simulink model "x35BusNetworkElectricityTransmissionModel"  (R2023b)
settings: Solver=VariableStepAuto  StartTime=0.0  StopTime=0.8  RelTol=1e-3
model workspace (MAT data in the model file):
  Compensation_Ki = 30
  Compensation_Kp = 3
  DC_Ki = 400
  DC_Kp = 8
  F = 0.01
  Flux_min = 0.5
  Grid_Freq_PWM = 2700
  Grid_Ireg_Ki = 5
  Grid_Ireg_Kp = 0.83
  Grid_Ireg_lim = 1.1
  Grid_Modindex_Upper = 1.1
  Grid_conv_Imax = 0.8
  H = 0.685
  Idref_max = 0.9
  Iqref_Tc = 0.3
  Ki_Var = 0.05
  Ki_Vreg = 20
  Ksh = 1.1
  L_pu = 0.3
  Llr = 0.16
  Lls = 0.18
  Lm = 2.9
  Nb_wt = 6
  P_mech = 1080000
  Pitch_Ki = 0
  Pitch_Kp = 150
  Pitch_Max = 27
  Pitch_Tc = 0.01
  Pitch_rate = 10
  Q_Filt = 50
  R_pu = 0.003
  Rotor_Freq_PWM = 1620
  Rotor_Ireg_Ki = 8
  Rotor_Ireg_Kp = 0.6
  Rotor_Ireg_lim = 0.1
  Rotor_Modindex_Upper = 2
  Rr = 0.016
  Rs = 0.023
  T_set = 0.0001
  Tp = 5e-05
  Ts = 5e-06
  Var_C_Filt = 720000
  Var_reg_max = 1.1
  Var_reg_min = 0.9
  WT_Coeff = [0.645 116 0.4 5 21 0.00912 0.08 0.035]
  WT_H = 4.32
  WT_IGBTRon = 5.931
  WT_Param = [91.204 10143]
  Wind_Freq_Filt = 10000
  Wind_Freq_nom = 60
  Wind_P_nom = 1200000
  Wind_Rotor_V_nom = 1950
  Wind_V_nom = 500
  Zeta_Filt = 0.707106781187
  init = [-0.2 0 0 0 0 0 0 0]
  p = 3
  torque0 = 0.83
  v_Ki = 0.1
  v_Kp = 3.6
  v_Max = 1.2
  v_Min = 0.7
  v_T = 5
  vreg_max = 1
  wind_VDC_nom = 1150
  wt0 = 1.2
undefined symbols (not defined in the file): D1, D11, Delta, DiscIntNeverNeededParam, Ion, Lithium, P, Q
libraries: powerlib_extras x144, spsSeriesRLCBranchLib x67, spsLoadFlowBusLib x43, spsThreePhaseTransformerTwoWindingsLib x32, spsThreePhaseSeriesRLCLoadLib x31, spsThreePhaseVIMeasurementLib x26, simulink_extras x26, spsDistributedParametersLineLib x22, spsGenericPowerSystemStabilizerLib x20, spsSynchronousMachinepuStandardLib x10, spsExcitationSystemLib x10, spsHydraulicTurbineandGovernorLib x10
(part 9 of 16)

== system x35BusNetworkElectricityTransmissionModel/ 41.4 MW Wind Generation/41.4 MW Wind Farm/Control System/Control System 4 ==
  Vabc : Inport
  Stator_Iabc : Inport  Port=2
  Grid_Iabc : Inport  Port=3
  Rotor_Iabc : Inport  Port=4
  Vdc_V : Inport  Port=5
  Qref1 : Inport  Port=6
  angle_rotor_rad : Inport  Port=7
  wr : Inport  Port=8
  Bus Creator : BusCreator  Inputs=P,Q
  Constant : Constant  Value=0
  Grid-side Control System : Subsystem
  "Measurement and abc-to-dq transformation " : Subsystem
  PWM Generator (2-Level) : spsPWMGenerator2LevelLib/PWM Generator (2-Level)  ModulatorType=Three-phase bridge (6 pulses)  ModulatorMode=Unsynchronized  Fc=Grid_Freq_PWM  Pc=90  nF=27  MinMax="[ -1  1 ]"  SamplingTechnique=Natural  ModulatingSignals=off  m=0.8  Freq=60  Phase=0  Ts=Ts  ShowCarrierOutport=off
  PWM Generator (2-Level)1 : spsPWMGenerator2LevelLib/PWM Generator (2-Level)  ModulatorType=Three-phase bridge (6 pulses)  ModulatorMode=Unsynchronized  Fc=Rotor_Freq_PWM  Pc=90  nF=27  MinMax="[ -1  1 ]"  SamplingTechnique=Natural  ModulatingSignals=off  m=0.8  Freq=60  Phase=0  Ts=Ts  ShowCarrierOutport=off
  Rotor-side Control System : Subsystem
  Speed & Pitch Control System : Subsystem
  Unit Delay{,2..5} (5 alike) : UnitDelay  SampleTime=Ts  HasFrameUpgradeWarning=on
  Grid_conv_pulses : Outport
  Rotor_conv_pulses : Outport  Port=2
  Pitch : Outport  Port=3
  PQ : Outport  Port=4
  wires:
  [Meas_P] -> Speed & Pitch Control System/2(Meas_P)
  "Measurement and abc-to-dq transformation "/1(Stator_Vdq) -> [Stator_Vdq]
  [Meas_Q] -> Unit Delay4/1
  Unit Delay4/1 -> Bus Creator/2  "Q"
  "Measurement and abc-to-dq transformation "/2(Stator_Idq) -> [Stator_Idq]
  "Measurement and abc-to-dq transformation "/9(w) -> [w]
  Grid_Iabc/1 -> "Measurement and abc-to-dq transformation "/3(Grid_Iabc)
  Grid-side Control System/1(Grid_conv_V) -> Unit Delay/1
  Unit Delay5/1 -> PWM Generator (2-Level)1/1
  Unit Delay2/1 -> Pitch/1
  Unit Delay/1 -> PWM Generator (2-Level)/1
  "Measurement and abc-to-dq transformation "/3(Grid_conv_Idq) -> [Grid_Idq]
  Rotor-side Control System/1(Uctrl_rotor_conv) -> Unit Delay5/1
  "Measurement and abc-to-dq transformation "/13(Delta_Rotor_Angle) -> [Delta_rotor_angle]
  PWM Generator (2-Level)/1 -> Grid_conv_pulses/1
  Vabc/1 -> "Measurement and abc-to-dq transformation "/1(Vabc)
  PWM Generator (2-Level)1/1 -> Rotor_conv_pulses/1
  "Measurement and abc-to-dq transformation "/4(Rotor_Idq) -> [Rotor_Idq]
  "Measurement and abc-to-dq transformation "/5(Vdc_meas_V) -> [Meas_VDC]
  angle_rotor_rad/1 -> "Measurement and abc-to-dq transformation "/7(angle_rotor_rad)
  wr/1 -> "Measurement and abc-to-dq transformation "/8(wr)
  "Measurement and abc-to-dq transformation "/7(Meas_Q) -> [Meas_Q]
  Speed & Pitch Control System/2(Pitch (deg)) -> Unit Delay2/1
  Stator_Iabc/1 -> "Measurement and abc-to-dq transformation "/2(Stator_Iabc)
  Speed & Pitch Control System/1(Tem_cmd) -> [Tem_cmd]
  Rotor_Iabc/1 -> "Measurement and abc-to-dq transformation "/4(Rotor_Iabc)
  Vdc_V/1 -> "Measurement and abc-to-dq transformation "/5(Vdc_V)
  Qref1/1 -> "Measurement and abc-to-dq transformation "/6(Qref)
  [wr] -> Speed & Pitch Control System/1(wr1)
  [Meas_P] -> Unit Delay3/1
  Unit Delay3/1 -> Bus Creator/1  "P"
  "Measurement and abc-to-dq transformation "/11("Qref ") -> [Q_ref]
  "Measurement and abc-to-dq transformation "/6(Meas_P) -> [Meas_P]
  "Measurement and abc-to-dq transformation "/12(Theta_PLL) -> [PLL_theta]
  Bus Creator/1 -> PQ/1
  "Measurement and abc-to-dq transformation "/8(Meas_V) -> [Meas_V]
  "Measurement and abc-to-dq transformation "/10("wr ") -> [wr]
  [Stator_Vdq] -> Grid-side Control System/1(Stator_Vdq)
  Constant/1 -> Grid-side Control System/2(Iq_ref)
  [Meas_VDC] -> Grid-side Control System/3(Vdc)
  [Grid_Idq] -> Grid-side Control System/4(Grid_conv_Idq)
  [PLL_theta] -> Grid-side Control System/5(Theta_PLL)
  [w] -> Grid-side Control System/6(w)
  [Rotor_Idq] -> Rotor-side Control System/1(Rotor_Idq)
  [wr] -> Rotor-side Control System/2(wr)
  [Meas_VDC] -> Rotor-side Control System/3(Vdc)
  [Delta_rotor_angle] -> Rotor-side Control System/4(Angle)
  [Q_ref] -> Rotor-side Control System/5(Qref)
  [Meas_Q] -> Rotor-side Control System/6(Meas_Q)
  [Meas_V] -> Rotor-side Control System/7(Meas_V)
  [Stator_Vdq] -> Rotor-side Control System/8(Stator_Vdq)
  [w] -> Rotor-side Control System/9(w)
  [Stator_Idq] -> Rotor-side Control System/10(Stator_Idq)
  [Tem_cmd] -> Rotor-side Control System/11(Tem_cmd)

== system x35BusNetworkElectricityTransmissionModel/400 kV Solar Farm/DC//DC Boost Converter/MPPT/MPPT  ==
  note: This model uses incremental conductance method to get maximum power point
      |
      | when dP/dV=0  where P= V*I
      | -> d(V*I)/dV = I + V*dI/dV = 0
      | -> dI/dV = -I/V
      |
      | The integrator functions to reduce/minimize errors (dI/dV + I/V)
      | Output = duty cycle changes
  PV_Current : Inport
  PV_Voltage : Inport  Port=2
  Switch port : Inport  Port=3
  Constant2 : Constant  Value=0
  Constant3 : Constant  Value=0
  Dead Zone : DeadZone  LowerValue=-0.05  UpperValue=0.05
  Discrete-Time Integrator : DiscreteIntegrator  SampleTime=T_set  LimitOutput=on  UpperSaturationLimit=1  LowerSaturationLimit=-1  ICPrevOutput=DiscIntNeverNeededParam  ICPrevScaledInput=DiscIntNeverNeededParam
  Fourier : spsFourierLib/Fourier  Freq=1/(MPPT_time)  n=1  InInit=[0, 0]  Ts=T_set
  Fourier1 : spsFourierLib/Fourier  Freq=1/(MPPT_time)  n=1  InInit=[0, 0]  Ts=T_set
  Gain : Gain  Gain=5
  Mean : spsMeanLib/Mean  Freq=1/(MPPT_time)  Vinit=0  Ts=T_set
  Mean1 : spsMeanLib/Mean  Freq=1/(MPPT_time)  Vinit=0  Ts=T_set
  Product : Product  Inputs=*/
  Product2 : Product
  Product3 : Product  Inputs=*/
  Saturation : Saturate  UpperLimit=inf  LowerLimit=eps  ZeroCross=off
  Saturation1 : Saturate  UpperLimit=inf  LowerLimit=eps  ZeroCross=off
  Sum : Sum  Inputs=+-
  Sum1 : Sum
  Switch : Switch  Threshold=0.5  SaturateOnIntegerOverflow=off  InputSameDT=off
  Switch1 : Switch  Threshold=0.5  SaturateOnIntegerOverflow=off  InputSameDT=off
  Trigonometric Function : Trigonometry  Operator=cos
  deg-to-rad conversion : Gain  Gain=pi/180
  delta D : Outport
  tag scope: Imean_PV1=global, Vmean_PV1=global
  wires:
  Mean1/1 -> [Vmean_PV1], Saturation1/1
  PV_Voltage/1 -> Mean1/1, Fourier1/1
  Sum/1 -> deg-to-rad conversion/1
  Product/1 -> Product2/1
  Product3/1 -> Sum1/2
  Saturation1/1 -> Product3/2
  Switch port/1 -> Switch/2, Switch1/2
  Mean/1 -> [Imean_PV1], Product3/1
  Dead Zone/1 -> Gain/1
  Fourier/2 -> Sum/1
  Fourier1/1 -> Saturation/1
  Sum1/1 -> Switch/1  "error"
  Constant2/1 -> Switch/3
  Trigonometric Function/1 -> Product2/2
  Gain/1 -> Discrete-Time Integrator/1
  Discrete-Time Integrator/1 -> Switch1/1
  Switch/1 -> Dead Zone/1
  Fourier1/2 -> Sum/2
  Constant3/1 -> Switch1/3
  deg-to-rad conversion/1 -> Trigonometric Function/1
  PV_Current/1 -> Mean/1, Fourier/1
  Product2/1 -> Sum1/1  "dI/dV (PV)"
  Saturation/1 -> Product/2
  Fourier/1 -> Product/1
  Switch1/1 -> delta D/1

== system x35BusNetworkElectricityTransmissionModel/400 kV Solar Farm/DC//DC Boost Converter1/MPPT/MPPT  ==
  note: This model uses incremental conductance method to get maximum power point
      |
      | when dP/dV=0  where P= V*I
      | -> d(V*I)/dV = I + V*dI/dV = 0
      | -> dI/dV = -I/V
      |
      | The integrator functions to reduce/minimize errors (dI/dV + I/V)
      | Output = duty cycle changes
  PV_Current : Inport
  PV_Voltage : Inport  Port=2
  Switch port : Inport  Port=3
  Constant2 : Constant  Value=0
  Constant3 : Constant  Value=0
  Dead Zone : DeadZone  LowerValue=-0.05  UpperValue=0.05
  Discrete-Time Integrator : DiscreteIntegrator  SampleTime=T_set  LimitOutput=on  UpperSaturationLimit=1  LowerSaturationLimit=-1  ICPrevOutput=DiscIntNeverNeededParam  ICPrevScaledInput=DiscIntNeverNeededParam
  Fourier : spsFourierLib/Fourier  Freq=1/(MPPT_time)  n=1  InInit=[0, 0]  Ts=T_set
  Fourier1 : spsFourierLib/Fourier  Freq=1/(MPPT_time)  n=1  InInit=[0, 0]  Ts=T_set
  Gain : Gain  Gain=5
  Mean : spsMeanLib/Mean  Freq=1/(MPPT_time)  Vinit=0  Ts=T_set
  Mean1 : spsMeanLib/Mean  Freq=1/(MPPT_time)  Vinit=0  Ts=T_set
  Product : Product  Inputs=*/
  Product2 : Product
  Product3 : Product  Inputs=*/
  Saturation : Saturate  UpperLimit=inf  LowerLimit=eps  ZeroCross=off
  Saturation1 : Saturate  UpperLimit=inf  LowerLimit=eps  ZeroCross=off
  Sum : Sum  Inputs=+-
  Sum1 : Sum
  Switch : Switch  Threshold=0.5  SaturateOnIntegerOverflow=off  InputSameDT=off
  Switch1 : Switch  Threshold=0.5  SaturateOnIntegerOverflow=off  InputSameDT=off
  Trigonometric Function : Trigonometry  Operator=cos
  deg-to-rad conversion : Gain  Gain=pi/180
  delta D : Outport
  tag scope: Imean_PV2=global, Vmean_PV2=global
  wires:
  Mean1/1 -> Saturation1/1
  PV_Voltage/1 -> Mean1/1, Fourier1/1
  Sum/1 -> deg-to-rad conversion/1
  Product/1 -> Product2/1
  Product3/1 -> Sum1/2
  Saturation1/1 -> [Vmean_PV2], Product3/2
  Switch port/1 -> Switch/2, Switch1/2
  Mean/1 -> [Imean_PV2], Product3/1
  Dead Zone/1 -> Gain/1
  Fourier/2 -> Sum/1
  Fourier1/1 -> Saturation/1
  Sum1/1 -> Switch/1  "error"
  Constant2/1 -> Switch/3
  Trigonometric Function/1 -> Product2/2
  Gain/1 -> Discrete-Time Integrator/1
  Discrete-Time Integrator/1 -> Switch1/1
  Switch/1 -> Dead Zone/1
  Fourier1/2 -> Sum/2
  Constant3/1 -> Switch1/3
  deg-to-rad conversion/1 -> Trigonometric Function/1
  PV_Current/1 -> Mean/1, Fourier/1
  Product2/1 -> Sum1/1  "dI/dV (PV)"
  Saturation/1 -> Product/2
  Fourier/1 -> Product/1
  Switch1/1 -> delta D/1

== system x35BusNetworkElectricityTransmissionModel/400 kV Solar Farm/DC//DC Boost Converter2/MPPT/MPPT  ==
  note: This model uses incremental conductance method to get maximum power point
      |
      | when dP/dV=0  where P= V*I
      | -> d(V*I)/dV = I + V*dI/dV = 0
      | -> dI/dV = -I/V
      |
      | The integrator functions to reduce/minimize errors (dI/dV + I/V)
      | Output = duty cycle changes
  PV_Current : Inport
  PV_Voltage : Inport  Port=2
  Switch port : Inport  Port=3
  Constant2 : Constant  Value=0
  Constant3 : Constant  Value=0
  Dead Zone : DeadZone  LowerValue=-0.05  UpperValue=0.05
  Discrete-Time Integrator : DiscreteIntegrator  SampleTime=T_set  LimitOutput=on  UpperSaturationLimit=1  LowerSaturationLimit=-1  ICPrevOutput=DiscIntNeverNeededParam  ICPrevScaledInput=DiscIntNeverNeededParam
  Display : Display
  Fourier : spsFourierLib/Fourier  Freq=1/(MPPT_time)  n=1  InInit=[0, 0]  Ts=T_set
  Fourier1 : spsFourierLib/Fourier  Freq=1/(MPPT_time)  n=1  InInit=[0, 0]  Ts=T_set
  Gain : Gain  Gain=5
  Mean : spsMeanLib/Mean  Freq=1/(MPPT_time)  Vinit=0  Ts=T_set
  Mean1 : spsMeanLib/Mean  Freq=1/(MPPT_time)  Vinit=0  Ts=T_set
  Product : Product  Inputs=*/
  Product2 : Product
  Product3 : Product  Inputs=*/
  Saturation : Saturate  UpperLimit=inf  LowerLimit=eps  ZeroCross=off
  Saturation1 : Saturate  UpperLimit=inf  LowerLimit=eps  ZeroCross=off
  Sum : Sum  Inputs=+-
  Sum1 : Sum
  Switch : Switch  Threshold=0.5  SaturateOnIntegerOverflow=off  InputSameDT=off
  Switch1 : Switch  Threshold=0.5  SaturateOnIntegerOverflow=off  InputSameDT=off
  Trigonometric Function : Trigonometry  Operator=cos
  deg-to-rad conversion : Gain  Gain=pi/180
  delta D : Outport
  tag scope: Imean_PV3=global, Vmean_PV3=global
  wires:
  Mean1/1 -> Saturation1/1
  PV_Voltage/1 -> Mean1/1, Fourier1/1
  Sum/1 -> deg-to-rad conversion/1
  Product/1 -> Product2/1
  Product3/1 -> Sum1/2
  Saturation1/1 -> [Vmean_PV3], Product3/2
  Switch port/1 -> Switch/2, Switch1/2
  Dead Zone/1 -> Gain/1
  Fourier/2 -> Sum/1
  Fourier1/1 -> Saturation/1
  Sum1/1 -> Switch/1  "error"
  Constant2/1 -> Switch/3
  Trigonometric Function/1 -> Product2/2
  Gain/1 -> Discrete-Time Integrator/1
  Discrete-Time Integrator/1 -> Switch1/1
  Switch/1 -> Dead Zone/1
  Fourier1/2 -> Sum/2
  Constant3/1 -> Switch1/3
  deg-to-rad conversion/1 -> Trigonometric Function/1
  PV_Current/1 -> Mean/1, Fourier/1
  Product2/1 -> Sum1/1  "dI/dV (PV)"
  Saturation/1 -> Product/2
  Fourier/1 -> Product/1
  Switch1/1 -> delta D/1
  Mean/1 -> Display/1, [Imean_PV3], Product3/1

== system x35BusNetworkElectricityTransmissionModel/400 kV Solar Farm/DC//DC Boost Converter3/MPPT/MPPT  ==
  note: This model uses incremental conductance method to get maximum power point
      |
      | when dP/dV=0  where P= V*I
      | -> d(V*I)/dV = I + V*dI/dV = 0
      | -> dI/dV = -I/V
      |
      | The integrator functions to reduce/minimize errors (dI/dV + I/V)
      | Output = duty cycle changes
  PV_Current : Inport
  PV_Voltage : Inport  Port=2
  Switch port : Inport  Port=3
  Constant2 : Constant  Value=0
  Constant3 : Constant  Value=0
  Dead Zone : DeadZone  LowerValue=-0.05  UpperValue=0.05
  Discrete-Time Integrator : DiscreteIntegrator  SampleTime=T_set  LimitOutput=on  UpperSaturationLimit=1  LowerSaturationLimit=-1  ICPrevOutput=DiscIntNeverNeededParam  ICPrevScaledInput=DiscIntNeverNeededParam
  Fourier : spsFourierLib/Fourier  Freq=1/(MPPT_time)  n=1  InInit=[0, 0]  Ts=T_set
  Fourier1 : spsFourierLib/Fourier  Freq=1/(MPPT_time)  n=1  InInit=[0, 0]  Ts=T_set
  Gain : Gain  Gain=5
  Mean : spsMeanLib/Mean  Freq=1/(MPPT_time)  Vinit=0  Ts=T_set
  Mean1 : spsMeanLib/Mean  Freq=1/(MPPT_time)  Vinit=0  Ts=T_set
  Product : Product  Inputs=*/
  Product2 : Product
  Product3 : Product  Inputs=*/
  Saturation : Saturate  UpperLimit=inf  LowerLimit=eps  ZeroCross=off
  Saturation1 : Saturate  UpperLimit=inf  LowerLimit=eps  ZeroCross=off
  Sum : Sum  Inputs=+-
  Sum1 : Sum
  Switch : Switch  Threshold=0.5  SaturateOnIntegerOverflow=off  InputSameDT=off
  Switch1 : Switch  Threshold=0.5  SaturateOnIntegerOverflow=off  InputSameDT=off
  Trigonometric Function : Trigonometry  Operator=cos
  deg-to-rad conversion : Gain  Gain=pi/180
  delta D : Outport
  tag scope: Imean_PV4=global, Vmean_PV4=global
  wires:
  Mean1/1 -> Saturation1/1
  PV_Voltage/1 -> Mean1/1, Fourier1/1
  Sum/1 -> deg-to-rad conversion/1
  Product/1 -> Product2/1
  Product3/1 -> Sum1/2
  Saturation1/1 -> [Vmean_PV4], Product3/2
  Switch port/1 -> Switch/2, Switch1/2
  Dead Zone/1 -> Gain/1
  Fourier/2 -> Sum/1
  Fourier1/1 -> Saturation/1
  Sum1/1 -> Switch/1  "error"
  Constant2/1 -> Switch/3
  Trigonometric Function/1 -> Product2/2
  Gain/1 -> Discrete-Time Integrator/1
  Discrete-Time Integrator/1 -> Switch1/1
  Switch/1 -> Dead Zone/1
  Fourier1/2 -> Sum/2
  Constant3/1 -> Switch1/3
  deg-to-rad conversion/1 -> Trigonometric Function/1
  PV_Current/1 -> Mean/1, Fourier/1
  Product2/1 -> Sum1/1  "dI/dV (PV)"
  Saturation/1 -> Product/2
  Fourier/1 -> Product/1
  Switch1/1 -> delta D/1
  Mean/1 -> [Imean_PV4], Product3/1

== system x35BusNetworkElectricityTransmissionModel/North Network/Regulators 7/Turbine and Excitation Regulators/Stabilitator ==
  Pm : Inport
  Pe : Inport  Port=2
  dw : Inport  Port=3
  Add1 : Sum  Inputs=+-
  Generic Power System Stabilizer : spsGenericPowerSystemStabilizerLib/Generic Power System Stabilizer  Tsensor=30e-3  K=20  Twashout=2  Tleadlag1=[50e-3 20e-3]  Tleadlag2=[3 5.4]  VSlimits=[-0.15 0.15]  Vinit=0  Plot_On=off  MagdB_On=on  FreqRange=logspace(-2,2,500)
      settings: LibrarySourceBlock=|
      | sps_lib/Electrical Machines/Synchronous Machine Control/Generic
      | Power System Stabilizer
  Generic Power System Stabilizer1 : spsGenericPowerSystemStabilizerLib/Generic Power System Stabilizer  Tsensor=30e-3  K=20  Twashout=2  Tleadlag1=[50e-3 20e-3]  Tleadlag2=[3 5.4]  VSlimits=[-0.15 0.15]  Vinit=0  Plot_On=off  MagdB_On=on  FreqRange=logspace(-2,2,500)
      settings: LibrarySourceBlock=|
      | sps_lib/Electrical Machines/Synchronous Machine Control/Generic
      | Power System Stabilizer
  Ground : Ground
  Multiport Switch : MultiPortSwitch  DiagnosticForDefault=None  SaturateOnIntegerOverflow=off  InputSameDT=off
  Out1 : Outport
  wires:
  Pm/1 -> Add1/1
  Generic Power System Stabilizer1/1 -> Multiport Switch/4
  Pe/1 -> Add1/2
  Add1/1 -> Generic Power System Stabilizer/1
  Generic Power System Stabilizer/1 -> Multiport Switch/3
  dw/1 -> Generic Power System Stabilizer1/1
  Ground/1 -> Multiport Switch/2
  [PSS_modes] -> Multiport Switch/1
  Multiport Switch/1 -> Out1/1

== system x35BusNetworkElectricityTransmissionModel/North Network/Regulators 8/Turbine and Excitation Regulators/Stabilitator ==
  Pm : Inport
  Pe : Inport  Port=2
  dw : Inport  Port=3
  Add1 : Sum  Inputs=+-
  Generic Power System Stabilizer : spsGenericPowerSystemStabilizerLib/Generic Power System Stabilizer  Tsensor=30e-3  K=20  Twashout=2  Tleadlag1=[50e-3 20e-3]  Tleadlag2=[3 5.4]  VSlimits=[-0.15 0.15]  Vinit=0  Plot_On=off  MagdB_On=on  FreqRange=logspace(-2,2,500)
      settings: LibrarySourceBlock=|
      | sps_lib/Electrical Machines/Synchronous Machine Control/Generic
      | Power System Stabilizer
  Generic Power System Stabilizer1 : spsGenericPowerSystemStabilizerLib/Generic Power System Stabilizer  Tsensor=30e-3  K=20  Twashout=2  Tleadlag1=[50e-3 20e-3]  Tleadlag2=[3 5.4]  VSlimits=[-0.15 0.15]  Vinit=0  Plot_On=off  MagdB_On=on  FreqRange=logspace(-2,2,500)
      settings: LibrarySourceBlock=|
      | sps_lib/Electrical Machines/Synchronous Machine Control/Generic
      | Power System Stabilizer
  Ground : Ground
  Multiport Switch : MultiPortSwitch  DiagnosticForDefault=None  SaturateOnIntegerOverflow=off  InputSameDT=off
  Out1 : Outport
  wires:
  Pm/1 -> Add1/1
  Generic Power System Stabilizer1/1 -> Multiport Switch/4
  Pe/1 -> Add1/2
  Add1/1 -> Generic Power System Stabilizer/1
  Generic Power System Stabilizer/1 -> Multiport Switch/3
  dw/1 -> Generic Power System Stabilizer1/1
  Ground/1 -> Multiport Switch/2
  [PSS_modes] -> Multiport Switch/1
  Multiport Switch/1 -> Out1/1

== system x35BusNetworkElectricityTransmissionModel/North Network/Regulators 9/Turbine and Excitation Regulators/Stabilitator ==
  Pm : Inport
  Pe : Inport  Port=2
  dw : Inport  Port=3
  Add1 : Sum  Inputs=+-
  Generic Power System Stabilizer : spsGenericPowerSystemStabilizerLib/Generic Power System Stabilizer  Tsensor=30e-3  K=20  Twashout=2  Tleadlag1=[50e-3 20e-3]  Tleadlag2=[3 5.4]  VSlimits=[-0.15 0.15]  Vinit=0  Plot_On=off  MagdB_On=on  FreqRange=logspace(-2,2,500)
      settings: LibrarySourceBlock=|
      | sps_lib/Electrical Machines/Synchronous Machine Control/Generic
      | Power System Stabilizer
  Generic Power System Stabilizer1 : spsGenericPowerSystemStabilizerLib/Generic Power System Stabilizer  Tsensor=30e-3  K=20  Twashout=2  Tleadlag1=[50e-3 20e-3]  Tleadlag2=[3 5.4]  VSlimits=[-0.15 0.15]  Vinit=0  Plot_On=off  MagdB_On=on  FreqRange=logspace(-2,2,500)
      settings: LibrarySourceBlock=|
      | sps_lib/Electrical Machines/Synchronous Machine Control/Generic
      | Power System Stabilizer
  Ground : Ground
  Multiport Switch : MultiPortSwitch  DiagnosticForDefault=None  SaturateOnIntegerOverflow=off  InputSameDT=off
  Stab : Outport
  wires:
  Pm/1 -> Add1/1
  Generic Power System Stabilizer1/1 -> Multiport Switch/4
  Pe/1 -> Add1/2
  Add1/1 -> Generic Power System Stabilizer/1
  Generic Power System Stabilizer/1 -> Multiport Switch/3
  dw/1 -> Generic Power System Stabilizer1/1
  Ground/1 -> Multiport Switch/2
  [PSS_modes] -> Multiport Switch/1
  Multiport Switch/1 -> Stab/1

== system x35BusNetworkElectricityTransmissionModel/South Network/Regulators 1/Turbine and Excitation Regulators/Stabilitator ==
  Pm : Inport
  Pe : Inport  Port=2
  dw : Inport  Port=3
  Add1 : Sum  Inputs=+-
  Generic Power System Stabilizer : spsGenericPowerSystemStabilizerLib/Generic Power System Stabilizer  Tsensor=30e-3  K=20  Twashout=2  Tleadlag1=[50e-3 20e-3]  Tleadlag2=[3 5.4]  VSlimits=[-0.15 0.15]  Vinit=0  Plot_On=off  MagdB_On=on  FreqRange=logspace(-2,2,500)
      settings: LibrarySourceBlock=|
      | sps_lib/Electrical Machines/Synchronous Machine Control/Generic
      | Power System Stabilizer
  Generic Power System Stabilizer1 : spsGenericPowerSystemStabilizerLib/Generic Power System Stabilizer  Tsensor=30e-3  K=20  Twashout=2  Tleadlag1=[50e-3 20e-3]  Tleadlag2=[3 5.4]  VSlimits=[-0.15 0.15]  Vinit=0  Plot_On=off  MagdB_On=on  FreqRange=logspace(-2,2,500)
      settings: LibrarySourceBlock=|
      | sps_lib/Electrical Machines/Synchronous Machine Control/Generic
      | Power System Stabilizer
  Ground : Ground
  Multiport Switch : MultiPortSwitch  DiagnosticForDefault=None  SaturateOnIntegerOverflow=off  InputSameDT=off
  Out1 : Outport
  wires:
  Pm/1 -> Add1/1
  Generic Power System Stabilizer1/1 -> Multiport Switch/4
  Pe/1 -> Add1/2
  Add1/1 -> Generic Power System Stabilizer/1
  Generic Power System Stabilizer/1 -> Multiport Switch/3
  dw/1 -> Generic Power System Stabilizer1/1
  Ground/1 -> Multiport Switch/2
  [PSS_modes] -> Multiport Switch/1
  Multiport Switch/1 -> Out1/1

== system x35BusNetworkElectricityTransmissionModel/South Network/Regulators 2/Turbine and Excitation Regulators/Stabilitator ==
  Pm : Inport
  Pe : Inport  Port=2
  dw : Inport  Port=3
  Add1 : Sum  Inputs=+-
  Generic Power System Stabilizer : spsGenericPowerSystemStabilizerLib/Generic Power System Stabilizer  Tsensor=30e-3  K=20  Twashout=2  Tleadlag1=[50e-3 20e-3]  Tleadlag2=[3 5.4]  VSlimits=[-0.15 0.15]  Vinit=0  Plot_On=off  MagdB_On=on  FreqRange=logspace(-2,2,500)
      settings: LibrarySourceBlock=|
      | sps_lib/Electrical Machines/Synchronous Machine Control/Generic
      | Power System Stabilizer
  Generic Power System Stabilizer1 : spsGenericPowerSystemStabilizerLib/Generic Power System Stabilizer  Tsensor=30e-3  K=20  Twashout=2  Tleadlag1=[50e-3 20e-3]  Tleadlag2=[3 5.4]  VSlimits=[-0.15 0.15]  Vinit=0  Plot_On=off  MagdB_On=on  FreqRange=logspace(-2,2,500)
      settings: LibrarySourceBlock=|
      | sps_lib/Electrical Machines/Synchronous Machine Control/Generic
      | Power System Stabilizer
  Ground : Ground
  Multiport Switch : MultiPortSwitch  DiagnosticForDefault=None  SaturateOnIntegerOverflow=off  InputSameDT=off
  Out1 : Outport
  wires:
  Pm/1 -> Add1/1
  Generic Power System Stabilizer1/1 -> Multiport Switch/4
  Pe/1 -> Add1/2
  Add1/1 -> Generic Power System Stabilizer/1
  Generic Power System Stabilizer/1 -> Multiport Switch/3
  dw/1 -> Generic Power System Stabilizer1/1
  Ground/1 -> Multiport Switch/2
  [PSS_modes] -> Multiport Switch/1
  Multiport Switch/1 -> Out1/1

== system x35BusNetworkElectricityTransmissionModel/South Network/Regulators 3/Turbine and Excitation Regulators/Stabilitator ==
  Pm : Inport
  Pe : Inport  Port=2
  dw : Inport  Port=3
  Add1 : Sum  Inputs=+-
  Generic Power System Stabilizer : spsGenericPowerSystemStabilizerLib/Generic Power System Stabilizer  Tsensor=30e-3  K=20  Twashout=2  Tleadlag1=[50e-3 20e-3]  Tleadlag2=[3 5.4]  VSlimits=[-0.15 0.15]  Vinit=0  Plot_On=off  MagdB_On=on  FreqRange=logspace(-2,2,500)
      settings: LibrarySourceBlock=|
      | sps_lib/Electrical Machines/Synchronous Machine Control/Generic
      | Power System Stabilizer
  Generic Power System Stabilizer1 : spsGenericPowerSystemStabilizerLib/Generic Power System Stabilizer  Tsensor=30e-3  K=20  Twashout=2  Tleadlag1=[50e-3 20e-3]  Tleadlag2=[3 5.4]  VSlimits=[-0.15 0.15]  Vinit=0  Plot_On=off  MagdB_On=on  FreqRange=logspace(-2,2,500)
      settings: LibrarySourceBlock=|
      | sps_lib/Electrical Machines/Synchronous Machine Control/Generic
      | Power System Stabilizer
  Ground : Ground
  Multiport Switch : MultiPortSwitch  DiagnosticForDefault=None  SaturateOnIntegerOverflow=off  InputSameDT=off
  Out1 : Outport
  wires:
  Pm/1 -> Add1/1
  Generic Power System Stabilizer1/1 -> Multiport Switch/4
  Pe/1 -> Add1/2
  Add1/1 -> Generic Power System Stabilizer/1
  Generic Power System Stabilizer/1 -> Multiport Switch/3
  dw/1 -> Generic Power System Stabilizer1/1
  Ground/1 -> Multiport Switch/2
  [PSS_modes] -> Multiport Switch/1
  Multiport Switch/1 -> Out1/1

== system x35BusNetworkElectricityTransmissionModel/South Network/Regulators 4/Turbine and Excitation Regulators/Stabilitator ==
  Pm : Inport
  Pe : Inport  Port=2
  dw : Inport  Port=3
  Add1 : Sum  Inputs=+-
  Generic Power System Stabilizer : spsGenericPowerSystemStabilizerLib/Generic Power System Stabilizer  Tsensor=30e-3  K=20  Twashout=2  Tleadlag1=[50e-3 20e-3]  Tleadlag2=[3 5.4]  VSlimits=[-0.15 0.15]  Vinit=0  Plot_On=off  MagdB_On=on  FreqRange=logspace(-2,2,500)
      settings: LibrarySourceBlock=|
      | sps_lib/Electrical Machines/Synchronous Machine Control/Generic
      | Power System Stabilizer
  Generic Power System Stabilizer1 : spsGenericPowerSystemStabilizerLib/Generic Power System Stabilizer  Tsensor=30e-3  K=20  Twashout=2  Tleadlag1=[50e-3 20e-3]  Tleadlag2=[3 5.4]  VSlimits=[-0.15 0.15]  Vinit=0  Plot_On=off  MagdB_On=on  FreqRange=logspace(-2,2,500)
      settings: LibrarySourceBlock=|
      | sps_lib/Electrical Machines/Synchronous Machine Control/Generic
      | Power System Stabilizer
  Ground : Ground
  Multiport Switch : MultiPortSwitch  DiagnosticForDefault=None  SaturateOnIntegerOverflow=off  InputSameDT=off
  Out1 : Outport
  wires:
  Pm/1 -> Add1/1
  Generic Power System Stabilizer1/1 -> Multiport Switch/4
  Pe/1 -> Add1/2
  Add1/1 -> Generic Power System Stabilizer/1
  Generic Power System Stabilizer/1 -> Multiport Switch/3
  dw/1 -> Generic Power System Stabilizer1/1
  Ground/1 -> Multiport Switch/2
  [PSS_modes] -> Multiport Switch/1
  Multiport Switch/1 -> Out1/1

== system x35BusNetworkElectricityTransmissionModel/South Network/Regulators 5/Turbine and Excitation Regulators/Stabilitator ==
  Pm : Inport
  Pe : Inport  Port=2
  dw : Inport  Port=3
  Add1 : Sum  Inputs=+-
  Generic Power System Stabilizer : spsGenericPowerSystemStabilizerLib/Generic Power System Stabilizer  Tsensor=30e-3  K=20  Twashout=2  Tleadlag1=[50e-3 20e-3]  Tleadlag2=[3 5.4]  VSlimits=[-0.15 0.15]  Vinit=0  Plot_On=off  MagdB_On=on  FreqRange=logspace(-2,2,500)
      settings: LibrarySourceBlock=|
      | sps_lib/Electrical Machines/Synchronous Machine Control/Generic
      | Power System Stabilizer
  Generic Power System Stabilizer1 : spsGenericPowerSystemStabilizerLib/Generic Power System Stabilizer  Tsensor=30e-3  K=20  Twashout=2  Tleadlag1=[50e-3 20e-3]  Tleadlag2=[3 5.4]  VSlimits=[-0.15 0.15]  Vinit=0  Plot_On=off  MagdB_On=on  FreqRange=logspace(-2,2,500)
      settings: LibrarySourceBlock=|
      | sps_lib/Electrical Machines/Synchronous Machine Control/Generic
      | Power System Stabilizer
  Ground : Ground
  Multiport Switch : MultiPortSwitch  DiagnosticForDefault=None  SaturateOnIntegerOverflow=off  InputSameDT=off
  Out1 : Outport
  wires:
  Pm/1 -> Add1/1
  Generic Power System Stabilizer1/1 -> Multiport Switch/4
  Pe/1 -> Add1/2
  Add1/1 -> Generic Power System Stabilizer/1
  Generic Power System Stabilizer/1 -> Multiport Switch/3
  dw/1 -> Generic Power System Stabilizer1/1
  Ground/1 -> Multiport Switch/2
  [PSS_modes] -> Multiport Switch/1
  Multiport Switch/1 -> Out1/1

== system x35BusNetworkElectricityTransmissionModel/South Network/Regulators 6/Turbine and Excitation Regulators/Stabilitator ==
  Pm : Inport
  Pe : Inport  Port=2
  dw : Inport  Port=3
  Add1 : Sum  Inputs=+-
  Generic Power System Stabilizer : spsGenericPowerSystemStabilizerLib/Generic Power System Stabilizer  Tsensor=30e-3  K=20  Twashout=2  Tleadlag1=[50e-3 20e-3]  Tleadlag2=[3 5.4]  VSlimits=[-0.15 0.15]  Vinit=0  Plot_On=off  MagdB_On=on  FreqRange=logspace(-2,2,500)
      settings: LibrarySourceBlock=|
      | sps_lib/Electrical Machines/Synchronous Machine Control/Generic
      | Power System Stabilizer
  Generic Power System Stabilizer1 : spsGenericPowerSystemStabilizerLib/Generic Power System Stabilizer  Tsensor=30e-3  K=20  Twashout=2  Tleadlag1=[50e-3 20e-3]  Tleadlag2=[3 5.4]  VSlimits=[-0.15 0.15]  Vinit=0  Plot_On=off  MagdB_On=on  FreqRange=logspace(-2,2,500)
      settings: LibrarySourceBlock=|
      | sps_lib/Electrical Machines/Synchronous Machine Control/Generic
      | Power System Stabilizer
  Ground : Ground
  Multiport Switch : MultiPortSwitch  DiagnosticForDefault=None  SaturateOnIntegerOverflow=off  InputSameDT=off
  Out1 : Outport
  wires:
  Pm/1 -> Add1/1
  Generic Power System Stabilizer1/1 -> Multiport Switch/4
  Pe/1 -> Add1/2
  Add1/1 -> Generic Power System Stabilizer/1
  Generic Power System Stabilizer/1 -> Multiport Switch/3
  dw/1 -> Generic Power System Stabilizer1/1
  Ground/1 -> Multiport Switch/2
  [PSS_modes] -> Multiport Switch/1
  Multiport Switch/1 -> Out1/1

== system x35BusNetworkElectricityTransmissionModel/ 41.4 MW Wind Generation/41.4 MW Wind Farm/10.35 MW Wind Turbine 1/Wind Turbine & Generator 1/Shaft ==
  Speed : Inport
  Discrete-Time Integrator1 : DiscreteIntegrator  InitialCondition=torque0/Ksh  SampleTime=Ts  ICPrevOutput=DiscIntNeverNeededParam  ICPrevScaledInput=DiscIntNeverNeededParam
  Mutual damping : Gain  Gain=1.5  SaturateOnIntegerOverflow=on  OutDataTypeStr=Inherit: Same as input  ParamDataTypeStr=Inherit: Same as input
  Stiffness : Gain  Gain=Ksh  SaturateOnIntegerOverflow=on  OutDataTypeStr=Inherit: Same as input  ParamDataTypeStr=Inherit: Same as input
  Sum2 : Sum  InputSameDT=on  SaturateOnIntegerOverflow=on  OutDataTypeStr=Inherit: Same as first input
  wbase : Gain  Gain=125.7  SaturateOnIntegerOverflow=on  OutDataTypeStr=Inherit: Same as input  ParamDataTypeStr=Inherit: Same as input
  T_shaft (pu) : Outport  VectorParamsAs1DForOutWhenUnconnected=off
  wires:
  Mutual damping/1 -> Sum2/2
  Stiffness/1 -> Sum2/1
  Sum2/1 -> T_shaft (pu)/1
  Speed/1 -> Mutual damping/1, wbase/1
  Discrete-Time Integrator1/1 -> Stiffness/1
  wbase/1 -> Discrete-Time Integrator1/1

== system x35BusNetworkElectricityTransmissionModel/ 41.4 MW Wind Generation/41.4 MW Wind Farm/10.35 MW Wind Turbine 1/Wind Turbine & Generator 1/Turbine ==
  T_wt (pu) : Inport
  T_shaft (pu) : Inport  Port=2
  Generator speed (pu) : Inport  Port=3
  1_2H_WT : Gain  Gain=1/(2*WT_H)  SaturateOnIntegerOverflow=on  OutDataTypeStr=Inherit: Same as input  ParamDataTypeStr=Inherit: Same as input
  Discrete-Time Integrator : DiscreteIntegrator  InitialCondition=wt0  SampleTime=Ts  ICPrevOutput=DiscIntNeverNeededParam  ICPrevScaledInput=DiscIntNeverNeededParam
  Sum : Sum  Inputs=+-  InputSameDT=on  SaturateOnIntegerOverflow=on  OutDataTypeStr=Inherit: Same as first input
  Sum1 : Sum  Inputs=+-  InputSameDT=on  SaturateOnIntegerOverflow=on  OutDataTypeStr=Inherit: Same as first input
  Turbine speed : Outport
  W_wt (pu) : Outport  Port=2  VectorParamsAs1DForOutWhenUnconnected=off
  wires:
  Sum1/1 -> Turbine speed/1
  Sum/1 -> 1_2H_WT/1
  Discrete-Time Integrator/1 -> W_wt (pu)/1, Sum1/1
  1_2H_WT/1 -> Discrete-Time Integrator/1
  T_wt (pu)/1 -> Sum/1
  T_shaft (pu)/1 -> Sum/2
  Generator speed (pu)/1 -> Sum1/2

== system x35BusNetworkElectricityTransmissionModel/ 41.4 MW Wind Generation/41.4 MW Wind Farm/10.35 MW Wind Turbine 1/Wind Turbine & Generator 1/Wind Turbine  ==
  Generator speed (pu)1 : Inport
  Pitch angle (deg) : Inport  Port=2
  Wind speed (m/s) : Inport  Port=3
  ->pu : Gain  Gain=1/Pmech_Out
  Avoid div. by zero : Saturate  UpperLimit=inf  LowerLimit=eps
  "Avoid div. by zero " : Saturate  UpperLimit=inf  LowerLimit=eps
  Fcn1 : Fcn  Expr=WT_Param(1)*u[2]/u[1]
  Fcn2 : Fcn  Expr=WT_Coeff8(1)*(WT_Coeff8(6)*u[1] + (-WT_Coeff8(4) - WT_Coeff8(3)*(2.5 + u[2]) + WT_Coeff8(2)*(1/(u[1] + WT_Coeff8(7)*(2.5 + u[2])) -WT_Coeff8(8)/(1 + (2.5 + u[2])^3)))/exp(WT_Coeff8(5)*(1/(u[1] + WT_Coeff8(7)*(2.5 + u[2])) - WT_Coeff8(8)/(1 + (2.5 + u[2])^3))))
  "K2*Cp*wind^3 " : Fcn  Expr=WT_Param(2)*u[1]^3*u[2]
  Mux : Mux  Inputs=2
  Mux1 : Mux  Inputs=2
  Mux2 : Mux  Inputs=2
  Product2 : Product  Inputs=*/  InputSameDT=on  SaturateOnIntegerOverflow=on  OutDataTypeStr=Inherit: Same as first input
  Tt (pu) : Outport  VectorParamsAs1DForOutWhenUnconnected=off
  wires:
  Generator speed (pu)1/1 -> "Avoid div. by zero "/1
  Mux1/1 -> Fcn2/1
  ->pu/1 -> Product2/1  "power_pu"
  Avoid div. by zero/1 -> Mux/1, Mux2/1
  "Avoid div. by zero "/1 -> Product2/2, Mux/2
  "K2*Cp*wind^3 "/1 -> ->pu/1
  Mux2/1 -> "K2*Cp*wind^3 "/1
  Fcn1/1 -> Mux1/1  "lambda"
  Mux/1 -> Fcn1/1
  Pitch angle (deg)/1 -> Mux1/2
  Wind speed (m/s)/1 -> Avoid div. by zero/1
  Product2/1 -> Tt (pu)/1
  Fcn2/1 -> Mux2/2  "Cp"

== system x35BusNetworkElectricityTransmissionModel/ 41.4 MW Wind Generation/41.4 MW Wind Farm/10.35 MW Wind Turbine 2/Wind Turbine & Generator 1/Shaft ==
  Speed : Inport
  Discrete-Time Integrator1 : DiscreteIntegrator  InitialCondition=torque0/Ksh  SampleTime=Ts  ICPrevOutput=DiscIntNeverNeededParam  ICPrevScaledInput=DiscIntNeverNeededParam
  Mutual damping : Gain  Gain=1.5  SaturateOnIntegerOverflow=on  OutDataTypeStr=Inherit: Same as input  ParamDataTypeStr=Inherit: Same as input
  Stiffness : Gain  Gain=Ksh  SaturateOnIntegerOverflow=on  OutDataTypeStr=Inherit: Same as input  ParamDataTypeStr=Inherit: Same as input
  Sum2 : Sum  InputSameDT=on  SaturateOnIntegerOverflow=on  OutDataTypeStr=Inherit: Same as first input
  wbase : Gain  Gain=125.7  SaturateOnIntegerOverflow=on  OutDataTypeStr=Inherit: Same as input  ParamDataTypeStr=Inherit: Same as input
  T_shaft (pu) : Outport  VectorParamsAs1DForOutWhenUnconnected=off
  wires:
  Mutual damping/1 -> Sum2/2
  Stiffness/1 -> Sum2/1
  Sum2/1 -> T_shaft (pu)/1
  Speed/1 -> Mutual damping/1, wbase/1
  Discrete-Time Integrator1/1 -> Stiffness/1
  wbase/1 -> Discrete-Time Integrator1/1

== system x35BusNetworkElectricityTransmissionModel/ 41.4 MW Wind Generation/41.4 MW Wind Farm/10.35 MW Wind Turbine 2/Wind Turbine & Generator 1/Turbine ==
  T_wt (pu) : Inport
  T_shaft (pu) : Inport  Port=2
  Generator speed (pu) : Inport  Port=3
  1_2H_WT : Gain  Gain=1/(2*WT_H)  SaturateOnIntegerOverflow=on  OutDataTypeStr=Inherit: Same as input  ParamDataTypeStr=Inherit: Same as input
  Discrete-Time Integrator : DiscreteIntegrator  InitialCondition=wt0  SampleTime=Ts  ICPrevOutput=DiscIntNeverNeededParam  ICPrevScaledInput=DiscIntNeverNeededParam
  Sum : Sum  Inputs=+-  InputSameDT=on  SaturateOnIntegerOverflow=on  OutDataTypeStr=Inherit: Same as first input
  Sum1 : Sum  Inputs=+-  InputSameDT=on  SaturateOnIntegerOverflow=on  OutDataTypeStr=Inherit: Same as first input
  Turbine speed : Outport
  W_wt (pu) : Outport  Port=2  VectorParamsAs1DForOutWhenUnconnected=off
  wires:
  Sum1/1 -> Turbine speed/1
  Sum/1 -> 1_2H_WT/1
  Discrete-Time Integrator/1 -> W_wt (pu)/1, Sum1/1
  1_2H_WT/1 -> Discrete-Time Integrator/1
  T_wt (pu)/1 -> Sum/1
  T_shaft (pu)/1 -> Sum/2
  Generator speed (pu)/1 -> Sum1/2

== system x35BusNetworkElectricityTransmissionModel/ 41.4 MW Wind Generation/41.4 MW Wind Farm/10.35 MW Wind Turbine 2/Wind Turbine & Generator 1/Wind Turbine  ==
  Generator speed (pu)1 : Inport
  Pitch angle (deg) : Inport  Port=2
  Wind speed (m/s) : Inport  Port=3
  ->pu : Gain  Gain=1/Pmech_Out
  Avoid div. by zero : Saturate  UpperLimit=inf  LowerLimit=eps
  "Avoid div. by zero " : Saturate  UpperLimit=inf  LowerLimit=eps
  Fcn1 : Fcn  Expr=WT_Param(1)*u[2]/u[1]
  Fcn2 : Fcn  Expr=WT_Coeff8(1)*(WT_Coeff8(6)*u[1] + (-WT_Coeff8(4) - WT_Coeff8(3)*(2.5 + u[2]) + WT_Coeff8(2)*(1/(u[1] + WT_Coeff8(7)*(2.5 + u[2])) -WT_Coeff8(8)/(1 + (2.5 + u[2])^3)))/exp(WT_Coeff8(5)*(1/(u[1] + WT_Coeff8(7)*(2.5 + u[2])) - WT_Coeff8(8)/(1 + (2.5 + u[2])^3))))
  "K2*Cp*wind^3 " : Fcn  Expr=WT_Param(2)*u[1]^3*u[2]
  Mux : Mux  Inputs=2
  Mux1 : Mux  Inputs=2
  Mux2 : Mux  Inputs=2
  Product2 : Product  Inputs=*/  InputSameDT=on  SaturateOnIntegerOverflow=on  OutDataTypeStr=Inherit: Same as first input
  Tt (pu) : Outport  VectorParamsAs1DForOutWhenUnconnected=off
  wires:
  Generator speed (pu)1/1 -> "Avoid div. by zero "/1
  Mux1/1 -> Fcn2/1
  ->pu/1 -> Product2/1  "power_pu"
  Avoid div. by zero/1 -> Mux/1, Mux2/1
  "Avoid div. by zero "/1 -> Product2/2, Mux/2
  "K2*Cp*wind^3 "/1 -> ->pu/1
  Mux2/1 -> "K2*Cp*wind^3 "/1
  Fcn1/1 -> Mux1/1  "lambda"
  Mux/1 -> Fcn1/1
  Pitch angle (deg)/1 -> Mux1/2
  Wind speed (m/s)/1 -> Avoid div. by zero/1
  Product2/1 -> Tt (pu)/1
  Fcn2/1 -> Mux2/2  "Cp"

== system x35BusNetworkElectricityTransmissionModel/ 41.4 MW Wind Generation/41.4 MW Wind Farm/10.35 MW Wind Turbine 3/Wind Turbine & Generator 1/Shaft ==
  Speed : Inport
  Discrete-Time Integrator1 : DiscreteIntegrator  InitialCondition=torque0/Ksh  SampleTime=Ts  ICPrevOutput=DiscIntNeverNeededParam  ICPrevScaledInput=DiscIntNeverNeededParam
  Mutual damping : Gain  Gain=1.5  SaturateOnIntegerOverflow=on  OutDataTypeStr=Inherit: Same as input  ParamDataTypeStr=Inherit: Same as input
  Stiffness : Gain  Gain=Ksh  SaturateOnIntegerOverflow=on  OutDataTypeStr=Inherit: Same as input  ParamDataTypeStr=Inherit: Same as input
  Sum2 : Sum  InputSameDT=on  SaturateOnIntegerOverflow=on  OutDataTypeStr=Inherit: Same as first input
  wbase : Gain  Gain=125.7  SaturateOnIntegerOverflow=on  OutDataTypeStr=Inherit: Same as input  ParamDataTypeStr=Inherit: Same as input
  T_shaft (pu) : Outport  VectorParamsAs1DForOutWhenUnconnected=off
  wires:
  Mutual damping/1 -> Sum2/2
  Stiffness/1 -> Sum2/1
  Sum2/1 -> T_shaft (pu)/1
  Speed/1 -> Mutual damping/1, wbase/1
  Discrete-Time Integrator1/1 -> Stiffness/1
  wbase/1 -> Discrete-Time Integrator1/1

== system x35BusNetworkElectricityTransmissionModel/ 41.4 MW Wind Generation/41.4 MW Wind Farm/10.35 MW Wind Turbine 3/Wind Turbine & Generator 1/Turbine ==
  T_wt (pu) : Inport
  T_shaft (pu) : Inport  Port=2
  Generator speed (pu) : Inport  Port=3
  1_2H_WT : Gain  Gain=1/(2*WT_H)  SaturateOnIntegerOverflow=on  OutDataTypeStr=Inherit: Same as input  ParamDataTypeStr=Inherit: Same as input
  Discrete-Time Integrator : DiscreteIntegrator  InitialCondition=wt0  SampleTime=Ts  ICPrevOutput=DiscIntNeverNeededParam  ICPrevScaledInput=DiscIntNeverNeededParam
  Sum : Sum  Inputs=+-  InputSameDT=on  SaturateOnIntegerOverflow=on  OutDataTypeStr=Inherit: Same as first input
  Sum1 : Sum  Inputs=+-  InputSameDT=on  SaturateOnIntegerOverflow=on  OutDataTypeStr=Inherit: Same as first input
  Turbine speed : Outport
  W_wt (pu) : Outport  Port=2  VectorParamsAs1DForOutWhenUnconnected=off
  wires:
  Sum1/1 -> Turbine speed/1
  Sum/1 -> 1_2H_WT/1
  Discrete-Time Integrator/1 -> W_wt (pu)/1, Sum1/1
  1_2H_WT/1 -> Discrete-Time Integrator/1
  T_wt (pu)/1 -> Sum/1
  T_shaft (pu)/1 -> Sum/2
  Generator speed (pu)/1 -> Sum1/2

== system x35BusNetworkElectricityTransmissionModel/ 41.4 MW Wind Generation/41.4 MW Wind Farm/10.35 MW Wind Turbine 3/Wind Turbine & Generator 1/Wind Turbine  ==
  Generator speed (pu)1 : Inport
  Pitch angle (deg) : Inport  Port=2
  Wind speed (m/s) : Inport  Port=3
  ->pu : Gain  Gain=1/Pmech_Out
  Avoid div. by zero : Saturate  UpperLimit=inf  LowerLimit=eps
  "Avoid div. by zero " : Saturate  UpperLimit=inf  LowerLimit=eps
  Fcn1 : Fcn  Expr=WT_Param(1)*u[2]/u[1]
  Fcn2 : Fcn  Expr=WT_Coeff8(1)*(WT_Coeff8(6)*u[1] + (-WT_Coeff8(4) - WT_Coeff8(3)*(2.5 + u[2]) + WT_Coeff8(2)*(1/(u[1] + WT_Coeff8(7)*(2.5 + u[2])) -WT_Coeff8(8)/(1 + (2.5 + u[2])^3)))/exp(WT_Coeff8(5)*(1/(u[1] + WT_Coeff8(7)*(2.5 + u[2])) - WT_Coeff8(8)/(1 + (2.5 + u[2])^3))))
  "K2*Cp*wind^3 " : Fcn  Expr=WT_Param(2)*u[1]^3*u[2]
  Mux : Mux  Inputs=2
  Mux1 : Mux  Inputs=2
  Mux2 : Mux  Inputs=2
  Product2 : Product  Inputs=*/  InputSameDT=on  SaturateOnIntegerOverflow=on  OutDataTypeStr=Inherit: Same as first input
  Tt (pu) : Outport  VectorParamsAs1DForOutWhenUnconnected=off
  wires:
  Generator speed (pu)1/1 -> "Avoid div. by zero "/1
  Mux1/1 -> Fcn2/1
  ->pu/1 -> Product2/1  "power_pu"
  Avoid div. by zero/1 -> Mux/1, Mux2/1
  "Avoid div. by zero "/1 -> Product2/2, Mux/2
  "K2*Cp*wind^3 "/1 -> ->pu/1
  Mux2/1 -> "K2*Cp*wind^3 "/1
  Fcn1/1 -> Mux1/1  "lambda"
  Mux/1 -> Fcn1/1
  Pitch angle (deg)/1 -> Mux1/2
  Wind speed (m/s)/1 -> Avoid div. by zero/1
  Product2/1 -> Tt (pu)/1
  Fcn2/1 -> Mux2/2  "Cp"

== system x35BusNetworkElectricityTransmissionModel/ 41.4 MW Wind Generation/41.4 MW Wind Farm/10.35 MW Wind Turbine 4/Wind Turbine & Generator 1/Shaft ==
  Speed : Inport
  Discrete-Time Integrator1 : DiscreteIntegrator  InitialCondition=torque0/Ksh  SampleTime=Ts  ICPrevOutput=DiscIntNeverNeededParam  ICPrevScaledInput=DiscIntNeverNeededParam
  Mutual damping : Gain  Gain=1.5  SaturateOnIntegerOverflow=on  OutDataTypeStr=Inherit: Same as input  ParamDataTypeStr=Inherit: Same as input
  Stiffness : Gain  Gain=Ksh  SaturateOnIntegerOverflow=on  OutDataTypeStr=Inherit: Same as input  ParamDataTypeStr=Inherit: Same as input
  Sum2 : Sum  InputSameDT=on  SaturateOnIntegerOverflow=on  OutDataTypeStr=Inherit: Same as first input
  wbase : Gain  Gain=125.7  SaturateOnIntegerOverflow=on  OutDataTypeStr=Inherit: Same as input  ParamDataTypeStr=Inherit: Same as input
  T_shaft (pu) : Outport  VectorParamsAs1DForOutWhenUnconnected=off
  wires:
  Mutual damping/1 -> Sum2/2
  Stiffness/1 -> Sum2/1
  Sum2/1 -> T_shaft (pu)/1
  Speed/1 -> Mutual damping/1, wbase/1
  Discrete-Time Integrator1/1 -> Stiffness/1
  wbase/1 -> Discrete-Time Integrator1/1

== system x35BusNetworkElectricityTransmissionModel/ 41.4 MW Wind Generation/41.4 MW Wind Farm/10.35 MW Wind Turbine 4/Wind Turbine & Generator 1/Turbine ==
  T_wt (pu) : Inport
  T_shaft (pu) : Inport  Port=2
  Generator speed (pu) : Inport  Port=3
  1_2H_WT : Gain  Gain=1/(2*WT_H)  SaturateOnIntegerOverflow=on  OutDataTypeStr=Inherit: Same as input  ParamDataTypeStr=Inherit: Same as input
  Discrete-Time Integrator : DiscreteIntegrator  InitialCondition=wt0  SampleTime=Ts  ICPrevOutput=DiscIntNeverNeededParam  ICPrevScaledInput=DiscIntNeverNeededParam
  Sum : Sum  Inputs=+-  InputSameDT=on  SaturateOnIntegerOverflow=on  OutDataTypeStr=Inherit: Same as first input
  Sum1 : Sum  Inputs=+-  InputSameDT=on  SaturateOnIntegerOverflow=on  OutDataTypeStr=Inherit: Same as first input
  Turbine speed : Outport
  W_wt (pu) : Outport  Port=2  VectorParamsAs1DForOutWhenUnconnected=off
  wires:
  Sum1/1 -> Turbine speed/1
  Sum/1 -> 1_2H_WT/1
  Discrete-Time Integrator/1 -> W_wt (pu)/1, Sum1/1
  1_2H_WT/1 -> Discrete-Time Integrator/1
  T_wt (pu)/1 -> Sum/1
  T_shaft (pu)/1 -> Sum/2
  Generator speed (pu)/1 -> Sum1/2

== system x35BusNetworkElectricityTransmissionModel/ 41.4 MW Wind Generation/41.4 MW Wind Farm/10.35 MW Wind Turbine 4/Wind Turbine & Generator 1/Wind Turbine  ==
  Generator speed (pu)1 : Inport
  Pitch angle (deg) : Inport  Port=2
  Wind speed (m/s) : Inport  Port=3
  ->pu : Gain  Gain=1/Pmech_Out
  Avoid div. by zero : Saturate  UpperLimit=inf  LowerLimit=eps
  "Avoid div. by zero " : Saturate  UpperLimit=inf  LowerLimit=eps
  Fcn1 : Fcn  Expr=WT_Param(1)*u[2]/u[1]
  Fcn2 : Fcn  Expr=WT_Coeff8(1)*(WT_Coeff8(6)*u[1] + (-WT_Coeff8(4) - WT_Coeff8(3)*(2.5 + u[2]) + WT_Coeff8(2)*(1/(u[1] + WT_Coeff8(7)*(2.5 + u[2])) -WT_Coeff8(8)/(1 + (2.5 + u[2])^3)))/exp(WT_Coeff8(5)*(1/(u[1] + WT_Coeff8(7)*(2.5 + u[2])) - WT_Coeff8(8)/(1 + (2.5 + u[2])^3))))
  "K2*Cp*wind^3 " : Fcn  Expr=WT_Param(2)*u[1]^3*u[2]
  Mux : Mux  Inputs=2
  Mux1 : Mux  Inputs=2
  Mux2 : Mux  Inputs=2
  Product2 : Product  Inputs=*/  InputSameDT=on  SaturateOnIntegerOverflow=on  OutDataTypeStr=Inherit: Same as first input
  Tt (pu) : Outport  VectorParamsAs1DForOutWhenUnconnected=off
  wires:
  Generator speed (pu)1/1 -> "Avoid div. by zero "/1
  Mux1/1 -> Fcn2/1
  ->pu/1 -> Product2/1  "power_pu"
  Avoid div. by zero/1 -> Mux/1, Mux2/1
  "Avoid div. by zero "/1 -> Product2/2, Mux/2
  "K2*Cp*wind^3 "/1 -> ->pu/1
  Mux2/1 -> "K2*Cp*wind^3 "/1
  Fcn1/1 -> Mux1/1  "lambda"
  Mux/1 -> Fcn1/1
  Pitch angle (deg)/1 -> Mux1/2
  Wind speed (m/s)/1 -> Avoid div. by zero/1
  Product2/1 -> Tt (pu)/1
  Fcn2/1 -> Mux2/2  "Cp"

== system x35BusNetworkElectricityTransmissionModel/ 41.4 MW Wind Generation/41.4 MW Wind Farm/Control System/Control System 1/Grid-side Control System ==
  note: Required value for modulation index "m" to obtain 1 pu generated voltage by the converter:
  note: m = Vnom * 2*sqrt(2/3) / Vdc
  note: Where Vnom = RMS ph-ph nominal voltage
  Stator_Vdq : Inport
  Iq_ref : Inport  Port=2
  Vdc : Inport  Port=3
  Grid_conv_Idq : Inport  Port=4
  Theta_PLL : Inport  Port=5
  w : Inport  Port=6
  Current Regulator : Subsystem
  Grid Voltage Converter : Subsystem
  Modulation : Subsystem
  VDC Regulator : Subsystem
  Grid_conv_V : Outport  VectorParamsAs1DForOutWhenUnconnected=off
  wires:
  Current Regulator/1(Grid_conv_Vd) -> Modulation/1(x)
  Current Regulator/2(Grid_conv_Vq) -> Modulation/2(y)
  Grid Voltage Converter/1(Grid_conv_V) -> Grid_conv_V/1
  Theta_PLL/1 -> Grid Voltage Converter/2(Theta_PLL)
  VDC Regulator/1(Out1) -> Current Regulator/2(In2)
  Iq_ref/1 -> VDC Regulator/1(Iq_ref)
  Grid_conv_Idq/1 -> Current Regulator/3(Grid_conv_Idq)
  Stator_Vdq/1 -> Current Regulator/1(Stator_Vdq)
  w/1 -> Current Regulator/4(w)
  Modulation/1(Vdq0) -> Grid Voltage Converter/1(dq0)
  Vdc/1 -> VDC Regulator/2(Vdc)
